simulink model "open_loop_model"  (R2019b)
settings: Solver=VariableStepAuto  StartTime=0.0  StopTime=400  RelTol=1e-3
libraries: simulink x1
settings Model: NumberOfSteps=100  SnapshotBufferSize=50  SnapshotInterval=50  Creator=Dell  LastModifiedBy=srikesh

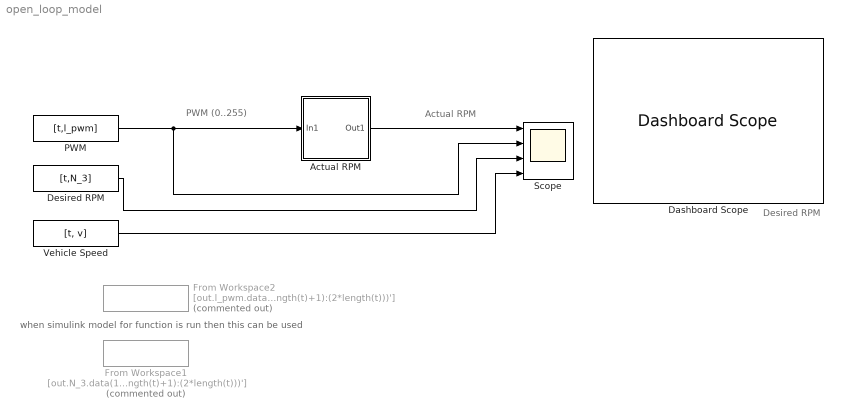
== system open_loop_model ==
  note: when simulink model for function is run then this can be used
  note: PWM (0..255)
  note: Desired RPM
  note: Actual RPM
  Actual RPM : Subsystem
  Dashboard Scope : DashboardScope
  Desired RPM : FromWorkspace  VariableName=[t,N_3]  SampleTime=0
  From Workspace1 : FromWorkspace  Commented=on  VariableName=[out.N_3.data(1:length(t))', out.N_3.data((length(t)+1):(2*length(t)))']  SampleTime=0
  From Workspace2 : FromWorkspace  Commented=on  VariableName=[out.l_pwm.data(1:length(t))', out.l_pwm.data((length(t)+1):(2*length(t)))']  SampleTime=0
  PWM : FromWorkspace  VariableName=[t,l_pwm]  SampleTime=0
  Scope : Scope  NumInputPorts=4
  "Vehicle Speed " : FromWorkspace  VariableName=[t, v]  SampleTime=0
  wires:
  Actual RPM/1(Out1) -> Scope/1
  PWM/1 -> Actual RPM/1(In1), Scope/2
  Desired RPM/1 -> Scope/3
  "Vehicle Speed "/1 -> Scope/4

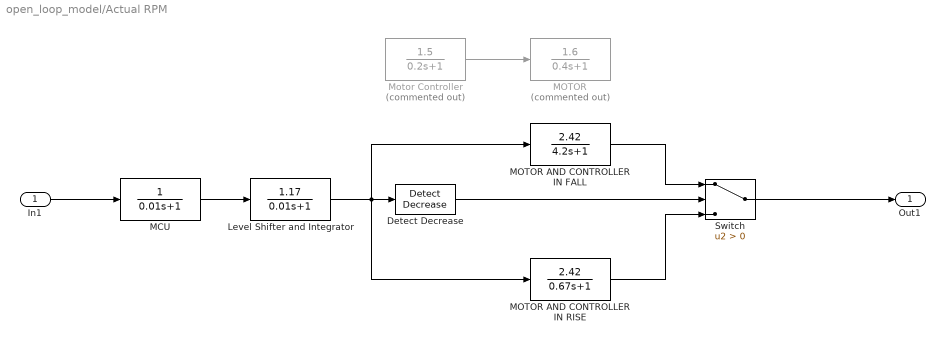
== system open_loop_model/Actual RPM ==
  In1 : Inport
  Detect Decrease : simulink/Logic and Bit Operations/Detect Decrease  vinit=0.0  OutDataTypeStr=boolean
  Level Shifter and Integrator : TransferFcn  Numerator=[1.17]  Denominator=[0.01 1]
  MCU : TransferFcn  Denominator=[0.01 1]
  MOTOR : TransferFcn  Commented=on  Numerator=[1.6]  Denominator=[0.4 1]
  MOTOR AND CONTROLLER IN FALL : TransferFcn  Numerator=[2.42]  Denominator=[4.2 1]
  MOTOR AND CONTROLLER IN RISE : TransferFcn  Numerator=[2.42]  Denominator=[0.67 1]
  Motor Controller : TransferFcn  Commented=on  Numerator=[1.5]  Denominator=[0.2 1]
  Switch : Switch  Criteria=u2 > Threshold
  Out1 : Outport
  wires:
  Motor Controller/1 -> MOTOR/1
  In1/1 -> MCU/1
  MCU/1 -> Level Shifter and Integrator/1
  Level Shifter and Integrator/1 -> MOTOR AND CONTROLLER IN RISE/1, MOTOR AND CONTROLLER IN FALL/1, Detect Decrease/1
  Detect Decrease/1 -> Switch/2
  MOTOR AND CONTROLLER IN FALL/1 -> Switch/1
  MOTOR AND CONTROLLER IN RISE/1 -> Switch/3
  Switch/1 -> Out1/1
